simulink model "momentumBasedFlying"  (Simulink 10.2)
settings: Solver=FixedStepAuto  StartTime=0.0  StopTime=Config.simulationTime  FixedStep=Config.tStep  RelTol=1e-3
InitFcn:
  | cd(fileparts(which(bdroot)));
  | initMomentumBasedFlying;
StopFcn:
  | cd(fileparts(which(bdroot)));
  | stopMomentumBasedFlying;
undefined symbols (not defined in the file or in its folder): biasVectorConstraint_feet, Config, confVisualizer, ConstraintMatrix_feet, DiscIntNeverNeededParam, jets_config
libraries: WBToolboxLibrary x85
(part 2 of 4)

== system momentumBasedFlying/FLYING CONTROLLER (CORE) V2.5/Flying State Machine/Compute Gains And References ==
  joyAxes : Inport
  joyButtons : Inport  Port=2
  systemState : Inport  Port=3
  jointPos : Inport  Port=4
  stateMachineQuantities : Inport  Port=5
  Bus Creator : BusCreator  Inputs=8
  "CoM6D ->  CoMXYZ5" : Selector  NumberOfDimensions=2  InputPortWidth=7  IndexOptions=Index vector (dialog),Index vector (dialog)  Indices=[1 2 3],[1]  OutputSizes=1,1
  Compute Gains : Subsystem
  Constant : Constant  Value=Config.references.gainSmoothingRotation
  Constant1 : Constant  Value=Config.references.smoothingTimeCoM
  Smooth CoM and Base References : Subsystem
  To Workspace : ToWorkspace  VariableName=posCoM_int  SaveFormat=Timeseries  SampleTime=-1
  Trajectory Generator : Subsystem
  holder 2 : WBToolboxLibrary/Utilities/holder 
      settings: SourceProductName=WholeBodyToolbox
  gainsAndReferences : Outport  VectorParamsAs1DForOutWhenUnconnected=off
  tag scope: jointPos_des=global, posCoM_des=global, rot_vel_acc_jerk_base_des=global
  wires:
  "CoM6D ->  CoMXYZ5"/1 -> [posCoM_des]
  Constant1/1 -> Smooth CoM and Base References/2(smoothingTimeCoMPos)
  Smooth CoM and Base References/2(rot_vel_acc_jerk_base_des_smooth) -> [rot_vel_acc_jerk_base_des], Bus Creator/2  "rot_vel_acc_jerk_base_des"
  Compute Gains/5(KP_torqueControl) -> Bus Creator/8  "KP_torqueControl"
  Compute Gains/2(KD_momentum) -> Bus Creator/5  "KD_momentum"
  Compute Gains/1(KP_momentum) -> Bus Creator/4  "KP_momentum"
  Compute Gains/3(KP_postural) -> Bus Creator/6  "KP_postural"
  Constant/1 -> Smooth CoM and Base References/3(gainSmoothingBaseRot)
  Bus Creator/1 -> gainsAndReferences/1
  Compute Gains/4(KI_torqueControl) -> Bus Creator/7  "KI_torqueControl"
  holder 2/1 -> Bus Creator/1, [jointPos_des]  "jointPos_des"
  jointPos/1 -> holder 2/1
  joyAxes/1 -> Trajectory Generator/1(joyAxes)
  joyButtons/1 -> Trajectory Generator/2(joyButtons)
  systemState/1 -> Trajectory Generator/3(systemState)
  stateMachineQuantities/1 -> Trajectory Generator/4(stateMachineQuantities)
  Trajectory Generator/1(pos_vel_acc_jerk_CoM_des) -> Smooth CoM and Base References/1(pos_vel_acc_jerk_CoM_des)
  Trajectory Generator/2(rot_vel_acc_jerk_base_des) -> Smooth CoM and Base References/4(rot_vel_acc_jerk_base_des)
  Trajectory Generator/3(posCoM_int) -> To Workspace/1
  Smooth CoM and Base References/1(pos_vel_acc_jerk_CoM_des_smooth) -> "CoM6D ->  CoMXYZ5"/1, Bus Creator/3  "pos_vel_acc_jerk_CoM_des"

== system momentumBasedFlying/FLYING CONTROLLER (CORE) V2.5/Flying State Machine/Take Off/Landing State Detector ==
  systemState : Inport
  joyButtons : Inport  Port=2
  Bus Creator : BusCreator  Inputs=6
  Bus Selector : BusSelector  OutputSignals=contactForces
  Demux : Demux  Outputs=[6;6]
  MATLAB Function : MATLAB Function  TreatAsAtomicUnit=on
  Vertical Forces Control : MATLAB Function  TreatAsAtomicUnit=on
  stateMachineQuantities : Outport  VectorParamsAs1DForOutWhenUnconnected=off
  tag scope: stateMachineQuantities=global
  wires:
  Vertical Forces Control/1(decreaseMaxFootVerticalForce) -> Bus Creator/1  "decreaseMaxFootVerticalForce"
  Vertical Forces Control/2(increaseMinFootVerticalForce) -> Bus Creator/2  "increaseMinFootVerticalForce"
  Bus Creator/1 -> [stateMachineQuantities], stateMachineQuantities/1
  systemState/1 -> Bus Selector/1
  joyButtons/1 -> Vertical Forces Control/1(joyButtons)
  Demux/2 -> MATLAB Function/2(wrench_r)
  Demux/1 -> MATLAB Function/1(wrench_l)
  Bus Selector/1 -> Demux/1  "<contactForces>"
  MATLAB Function/1(feetContactIsActive) -> Bus Creator/4  "feetContactIsActive"
  MATLAB Function/2(robotIsLanded) -> Bus Creator/5  "robotIsLanded"
  MATLAB Function/3(oneFootIsInContact) -> Bus Creator/6  "oneFootIsInContact"
  Vertical Forces Control/3(activateEqConstrTorqueControl) -> Bus Creator/3  "activateEqConstrTorqueControl"

== system momentumBasedFlying/FLYING CONTROLLER (CORE) V2.5/Get System State/Change Contact Forces Representation ==
  jointPos : Inport
  w_H_b : Inport  Port=2
  contactForces_WBD : Inport  Port=3
  Change Contact Forces Representation : MATLAB Function  TreatAsAtomicUnit=on
  "CoM6D ->  CoMXYZ1" : Selector  NumberOfDimensions=2  InputPortWidth=7  IndexOptions=Index vector (dialog),Index vector (dialog)  Indices=[1 2 3],[1 2 3]  OutputSizes=1,1
  "CoM6D ->  CoMXYZ3" : Selector  NumberOfDimensions=2  InputPortWidth=7  IndexOptions=Index vector (dialog),Index vector (dialog)  Indices=[1 2 3],[1 2 3]  OutputSizes=1,1
  LFoot Pose : WBToolboxLibrary/Model/Kinematics/ForwardKinematics  frameName=Frames.LFOOT_FRAME
      settings: SourceProductName=WholeBodyToolbox
  Mux : Mux  Inputs=2
  RFoot Pose : WBToolboxLibrary/Model/Kinematics/ForwardKinematics  frameName=Frames.RFOOT_FRAME
      settings: SourceProductName=WholeBodyToolbox
  contactForces : Outport  VectorParamsAs1DForOutWhenUnconnected=off
  tag scope: wrench_LFoot=global, wrench_RFoot=global
  wires:
  contactForces_WBD/1 -> Change Contact Forces Representation/1(contactForces_WBD)
  RFoot Pose/1 -> "CoM6D ->  CoMXYZ3"/1
  "CoM6D ->  CoMXYZ3"/1 -> Change Contact Forces Representation/3(w_R_r_sole)
  LFoot Pose/1 -> "CoM6D ->  CoMXYZ1"/1
  "CoM6D ->  CoMXYZ1"/1 -> Change Contact Forces Representation/2(w_R_l_sole)
  w_H_b/1 -> LFoot Pose/1, RFoot Pose/1
  jointPos/1 -> LFoot Pose/2, RFoot Pose/2
  Change Contact Forces Representation/1(mixed_f_l_sole) -> [wrench_LFoot], Mux/1
  Change Contact Forces Representation/2(mixed_f_r_sole) -> [wrench_RFoot], Mux/2
  Mux/1 -> contactForces/1

== system momentumBasedFlying/Visualizer/Task and Base Frame Kinematics/Combine Rotations ==
  roll : Inport
  pitch : Inport  Port=2
  yaw : Inport  Port=3
  roll_des : Inport  Port=4
  pitch_des : Inport  Port=5
  yaw_des : Inport  Port=6
  Mux : Mux  Inputs=2
  Mux1 : Mux  Inputs=2
  Mux2 : Mux  Inputs=2
  Task rotation combined : Scope  NumInputPorts=3
  wires:
  yaw_des/1 -> Mux2/2
  pitch_des/1 -> Mux1/2
  pitch/1 -> Mux1/1
  roll/1 -> Mux/1
  yaw/1 -> Mux2/1
  roll_des/1 -> Mux/2
  Mux2/1 -> Task rotation combined/3
  Mux1/1 -> Task rotation combined/2
  Mux/1 -> Task rotation combined/1

== system momentumBasedFlying/iRonCub/Forward Dynamics/old_simulator_subsystem ==
  joints_torque : Inport
  systemState : Inport  Port=2
  jets_input : Inport  Port=3
  Bus Creator : BusCreator  Inputs=5
  Bus Selector : BusSelector  Commented=on  OutputSignals=M,h
  Bus Selector1 : BusSelector  OutputSignals=baseTwist,jointVelocity,J_LFoot,J_RFoot,JDot_LFoot_nu,JDot_RFoot_nu,w_H_LFoot,w_H_RFoot,w_R_b
  Compute generalized external wrench and jet thrust : Subsystem
  Dynamics and Kinematics : Subsystem
  MATLAB Function1 : MATLAB Function  TreatAsAtomicUnit=on
  State Integration : Subsystem
  state : Outport
  wrench_LFoot : Outport  Port=2
  wrench_RFoot : Outport  Port=3
  wires:
  State Integration/3(basePose_dot) -> Bus Creator/3
  Dynamics and Kinematics/2(kinematics) -> Compute generalized external wrench and jet thrust/1(kinematics), Bus Selector1/1  "kinematics"
  Bus Selector1/6 -> MATLAB Function1/10(JDot_nu_RFOOT)  "<JDot_RFoot_nu>"
  Bus Selector1/7 -> MATLAB Function1/11(H_LFOOT)  "<w_H_LFoot>"
  Bus Selector1/4 -> MATLAB Function1/8(JRight_frameJac)  "<J_RFoot>"
  Bus Selector1/3 -> MATLAB Function1/7(JLeft_frameJac)  "<J_LFoot>"
  MATLAB Function1/4(dot_v_b) -> State Integration/5(dot_v_b)
  Bus Selector1/2 -> MATLAB Function1/6("joints_velocity ")  "<jointVelocity>"
  Compute generalized external wrench and jet thrust/1(generalized_jet_wrench) -> MATLAB Function1/4(generalized_ext_wrench)
  Bus Creator/1 -> state/1  "state"
  State Integration/4("joints_velocity ") -> Bus Creator/4
  Dynamics and Kinematics/1(dynamics) -> Bus Selector/1
  joints_torque/1 -> MATLAB Function1/3(joints_torque)
  State Integration/2(joints_position) -> Bus Creator/2
  MATLAB Function1/8(wrench_left_foot) -> wrench_LFoot/1  "wrench_LFoot"
  jets_input/1 -> Compute generalized external wrench and jet thrust/2(jets_input)
  State Integration/1(w_H_b) -> Bus Creator/1
  Bus Selector1/8 -> MATLAB Function1/12(H_RFOOT)  "<w_H_RFoot>"
  systemState/1 -> Dynamics and Kinematics/1(systemState)
  Bus Selector1/9 -> State Integration/1(<w_R_b>)  "<w_R_b>"
  Compute generalized external wrench and jet thrust/2(jets_intensities) -> Bus Creator/5  "jet_intensities"
  MATLAB Function1/6(joint_acceleration) -> State Integration/7(joint_acceleration)
  MATLAB Function1/3(joints_velocity) -> State Integration/4(joints_velocity)
  MATLAB Function1/9(wrench_right_foot) -> wrench_RFoot/1  "wrench_RFoot"
  Bus Selector1/5 -> MATLAB Function1/9(JDot_nu_LFOOT)  "<JDot_LFoot_nu>"
  Bus Selector/1 -> MATLAB Function1/1(mass_matrix)  "<M>"
  MATLAB Function1/1(base_linear_velocity) -> State Integration/2(base_linear_velocity)
  Bus Selector/2 -> MATLAB Function1/2(bias_forces)  "<h>"
  MATLAB Function1/7(contact_detected) -> State Integration/8(contact_detected)
  MATLAB Function1/2(omega_b) -> State Integration/3(omega_b)
  Bus Selector1/1 -> MATLAB Function1/5(base_velocity)  "<baseTwist>"
  MATLAB Function1/5(dot_omega_b) -> State Integration/6(dot_omega_b)

== system momentumBasedFlying/FLYING CONTROLLER (CORE) V2.5/Dynamics and Kinematics/Dynamic Quantities/Compute Centroidal Inertia ==
  M : Inport
  w_H_b : Inport  Port=2
  posCoM : Inport  Port=3
  Compute Centroidal Inertia : MATLAB Function  TreatAsAtomicUnit=on
  Selector : Selector  NumberOfDimensions=2  InputPortWidth=3  IndexOptions=Index vector (dialog),Index vector (dialog)  Indices=[1 2 3],4  OutputSizes=1,1
  w_I_c : Outport  VectorParamsAs1DForOutWhenUnconnected=off
  wires:
  M/1 -> Compute Centroidal Inertia/1(M)
  w_H_b/1 -> Selector/1
  Selector/1 -> Compute Centroidal Inertia/3(posBase)
  posCoM/1 -> Compute Centroidal Inertia/2(posCoM)
  Compute Centroidal Inertia/1(w_I_c) -> w_I_c/1

== system momentumBasedFlying/FLYING CONTROLLER (CORE) V2.5/Dynamics and Kinematics/Dynamic Quantities/Momentum and CentroidalMomentum Matrix ==
  w_H_b : Inport
  jointPos : Inport  Port=2
  w_baseTwist : Inport  Port=3
  jointVel : Inport  Port=4
  CentroidalMomentum : WBToolboxLibrary/Model/Dynamics/CentroidalMomentum
      settings: SourceProductName=WholeBodyToolbox
  CentroidalMomentum Matrix iCub 23/25 DoFs : Subsystem
  L : Outport  VectorParamsAs1DForOutWhenUnconnected=off
  CMM : Outport  Port=2  VectorParamsAs1DForOutWhenUnconnected=off
  wires:
  w_baseTwist/1 -> CentroidalMomentum/3
  CentroidalMomentum/1 -> L/1
  w_H_b/1 -> CentroidalMomentum Matrix iCub 23/25 DoFs/1(w_H_b), CentroidalMomentum/1
  jointPos/1 -> CentroidalMomentum Matrix iCub 23/25 DoFs/2(jointPos), CentroidalMomentum/2
  jointVel/1 -> CentroidalMomentum/4
  CentroidalMomentum Matrix iCub 23/25 DoFs/1(CMM) -> CMM/1

== system momentumBasedFlying/FLYING CONTROLLER (CORE) V2.5/Dynamics and Kinematics/Kinematic Quantities/Compute Thrusts Axes and Arms ==
  posCoM : Inport
  w_H_b : Inport  Port=2
  jointPos : Inport  Port=3
  Pose Jet 1 : WBToolboxLibrary/Model/Kinematics/ForwardKinematics  frameName=Frames.JET1_FRAME
      settings: SourceProductName=WholeBodyToolbox
  Pose Jet 2 : WBToolboxLibrary/Model/Kinematics/ForwardKinematics  frameName=Frames.JET2_FRAME
      settings: SourceProductName=WholeBodyToolbox
  Pose Jet 3 : WBToolboxLibrary/Model/Kinematics/ForwardKinematics  frameName=Frames.JET3_FRAME
      settings: SourceProductName=WholeBodyToolbox
  Pose Jet 4 : WBToolboxLibrary/Model/Kinematics/ForwardKinematics  frameName=Frames.JET4_FRAME
      settings: SourceProductName=WholeBodyToolbox
  Thrust Axes and Arms : MATLAB Function  TreatAsAtomicUnit=on
  matrixOfJetsAxes : Outport  VectorParamsAs1DForOutWhenUnconnected=off
  matrixOfJetsArms : Outport  Port=2  VectorParamsAs1DForOutWhenUnconnected=off
  wires:
  Pose Jet 2/1 -> Thrust Axes and Arms/2(w_H_J2)
  jointPos/1 -> Pose Jet 1/2, Pose Jet 2/2, Pose Jet 3/2, Pose Jet 4/2
  Pose Jet 1/1 -> Thrust Axes and Arms/1(w_H_J1)
  Pose Jet 3/1 -> Thrust Axes and Arms/3(w_H_J3)
  Pose Jet 4/1 -> Thrust Axes and Arms/4(w_H_J4)
  Thrust Axes and Arms/1(matrixOfJetsAxes) -> matrixOfJetsAxes/1
  Thrust Axes and Arms/2(matrixOfJetsArms) -> matrixOfJetsArms/1
  w_H_b/1 -> Pose Jet 4/1, Pose Jet 3/1, Pose Jet 2/1, Pose Jet 1/1
  posCoM/1 -> Thrust Axes and Arms/5(posCoM)

== system momentumBasedFlying/FLYING CONTROLLER (CORE) V2.5/Flying Controller v2.5/Joint Torque Control for Flying/Integrate Joints Velocity error ==
  jointVel_err : Inport
  Constant : Constant  Value=zeros(Config.N_DOF,1)
  Discrete-Time Integrator1 : DiscreteIntegrator  InitialConditionSource=external  InitialCondition=zeros(Config.N_DOF,1)  SampleTime=-1  ICPrevOutput=DiscIntNeverNeededParam  ICPrevScaledInput=DiscIntNeverNeededParam
  jointPos_err : Outport  VectorParamsAs1DForOutWhenUnconnected=off
  tag scope: jointPos_err_integral=global
  wires:
  Discrete-Time Integrator1/1 -> jointPos_err/1, [jointPos_err_integral]
  jointVel_err/1 -> Discrete-Time Integrator1/1
  Constant/1 -> Discrete-Time Integrator1/2

== system momentumBasedFlying/FLYING CONTROLLER (CORE) V2.5/Flying Controller v2.5/Joint Torque Control for Flying/QP_torqueControl ==
  Hessian : Inport
  gradient : Inport  Port=2
  ConstraintMatrix_inequality : Inport  Port=3
  biasVectorConstraint_inequality : Inport  Port=4
  feetContactIsActive : Inport  Port=5
  Constant2 : Constant  Value=Config.sat.jointTorquesSaturation
  Level-2 MATLAB S-Function1 : M-S-Function  FunctionName=QP_flyingTorqueControl  Parameters=Config.N_DOF
  jointTorques_star : Outport  VectorParamsAs1DForOutWhenUnconnected=off
  exitFlagQP_torqueControl : Outport  Port=2  VectorParamsAs1DForOutWhenUnconnected=off
  wires:
  Hessian/1 -> Level-2 MATLAB S-Function1/1
  Level-2 MATLAB S-Function1/1 -> jointTorques_star/1
  gradient/1 -> Level-2 MATLAB S-Function1/2
  Level-2 MATLAB S-Function1/2 -> exitFlagQP_torqueControl/1
  Constant2/1 -> Level-2 MATLAB S-Function1/6
  ConstraintMatrix_inequality/1 -> Level-2 MATLAB S-Function1/3
  biasVectorConstraint_inequality/1 -> Level-2 MATLAB S-Function1/4
  feetContactIsActive/1 -> Level-2 MATLAB S-Function1/5

== system momentumBasedFlying/FLYING CONTROLLER (CORE) V2.5/Flying Controller v2.5/Joint Torque Control for Flying/Torque Derivative Saturation ==
  jointTorques_star : Inport
  Constant1 : Constant  Value=Config.tStep
  Constant2 : Constant  Value=Config.sat.jointTorquesDotMax
  Saturate Torque Derivative : MATLAB Function  TreatAsAtomicUnit=on
  "holder " : WBToolboxLibrary/Utilities/holder 
      settings: SourceProductName=WholeBodyToolbox
  jointTorques_star_sat : Outport  VectorParamsAs1DForOutWhenUnconnected=off
  wires:
  jointTorques_star/1 -> "holder "/1, Saturate Torque Derivative/1(u)
  Saturate Torque Derivative/1(uSat) -> jointTorques_star_sat/1
  "holder "/1 -> Saturate Torque Derivative/2(u_0)
  Constant1/1 -> Saturate Torque Derivative/3(tStep)
  Constant2/1 -> Saturate Torque Derivative/4(uDotMax)

== system momentumBasedFlying/FLYING CONTROLLER (CORE) V2.5/Flying Controller v2.5/Momentum Control for Flying/Feedback linearization ==
  jetState : Inport
  jetDerivatives_des : Inport  Port=2
  Bus Selector : BusSelector  OutputSignals=jetIntensitiesFiltered,jetDerivativesEst
  Discrete-Time Integrator : DiscreteIntegrator  SampleTime=Config.tStep  ICPrevOutput=DiscIntNeverNeededParam  ICPrevScaledInput=DiscIntNeverNeededParam
  Error : Scope
  MATLAB Function : MATLAB Function  TreatAsAtomicUnit=on
  jetDerivatives : Scope  NumInputPorts=3
  throttle : Outport  VectorParamsAs1DForOutWhenUnconnected=off
  wires:
  Bus Selector/1 -> MATLAB Function/1(jets)  "<jetIntensitiesFiltered>"
  MATLAB Function/1(throttle) -> jetDerivatives/1, throttle/1  "throttle"
  jetState/1 -> Bus Selector/1
  MATLAB Function/2(error) -> Error/1, Discrete-Time Integrator/1  "error"
  Bus Selector/2 -> jetDerivatives/3, MATLAB Function/2(jets_dot)  "<jetDerivativesEst>"
  Discrete-Time Integrator/1 -> MATLAB Function/4(integral_err)
  jetDerivatives_des/1 -> MATLAB Function/3(jets_dot_des), jetDerivatives/2

== system momentumBasedFlying/FLYING CONTROLLER (CORE) V2.5/Flying Controller v2.5/Momentum Control for Flying/Momentum Control ==
  contactForces_hat : Inport
  systemState : Inport  Port=2
  kinematics : Inport  Port=3
  dynamics : Inport  Port=4
  gainsAndReferences : Inport  Port=5
  stateMachineQuantitites : Inport  Port=6
  Bus Selector : BusSelector  OutputSignals=jointPos,w_baseTwist,jetsIntensities,contactForces
  Bus Selector1 : BusSelector  OutputSignals=J_jets,J_CoM,J_LFoot,J_RFoot,posCoM,w_R_b,w_H_LFoot,w_H_RFoot,matrixOfJetAxes,matrixOfJetsArms
  Bus Selector2 : BusSelector  OutputSignals=w_I_c,L,M,CMM
  Bus Selector3 : BusSelector  OutputSignals=pos_vel_acc_jerk_CoM_des,rot_vel_acc_jerk_base_des,jointPos_des,KP_momentum,KD_momentum,KP_postural
  Bus Selector4 : BusSelector  OutputSignals=feetContactIsActive,decreaseMaxFootVerticalForce,increaseMinFootVerticalForce,robotIsLanded
  "Flying Controller Momentum FCN " : MATLAB Function  TreatAsAtomicUnit=on
  HessianMatrixQP : Outport  VectorParamsAs1DForOutWhenUnconnected=off
  gVectorQP : Outport  Port=2  VectorParamsAs1DForOutWhenUnconnected=off
  lowerBoundQP : Outport  Port=3  VectorParamsAs1DForOutWhenUnconnected=off
  uppeBoundQP : Outport  Port=4  VectorParamsAs1DForOutWhenUnconnected=off
  tag scope: LDot_estimated=global, momentum_des=global, verifyAngMomAndInertia=global
  wires:
  systemState/1 -> Bus Selector/1
  Bus Selector3/3 -> "Flying Controller Momentum FCN "/20(jointPos_des)  "<jointPos_des>"
  Bus Selector1/3 -> "Flying Controller Momentum FCN "/6(J_LFoot)  "<J_LFoot>"
  kinematics/1 -> Bus Selector1/1
  Bus Selector/1 -> "Flying Controller Momentum FCN "/1(jointPos)  "<jointPos>"
  Bus Selector1/1 -> "Flying Controller Momentum FCN "/4(J_jets)  "<J_jets>"
  Bus Selector/2 -> "Flying Controller Momentum FCN "/2(w_baseTwist)  "<w_baseTwist>"
  "Flying Controller Momentum FCN "/1(HessianMatrixQP) -> HessianMatrixQP/1
  "Flying Controller Momentum FCN "/4(upperBoundQP) -> uppeBoundQP/1
  "Flying Controller Momentum FCN "/2(gVectorQP) -> gVectorQP/1
  Bus Selector4/1 -> "Flying Controller Momentum FCN "/24(feetContactIsActive)  "<feetContactIsActive>"
  "Flying Controller Momentum FCN "/7(verifyAngMomAndInertia) -> [verifyAngMomAndInertia]
  stateMachineQuantitites/1 -> Bus Selector4/1
  "Flying Controller Momentum FCN "/3(lowerBoundQP) -> lowerBoundQP/1
  Bus Selector3/4 -> "Flying Controller Momentum FCN "/21(KP_momentum)  "<KP_momentum>"
  dynamics/1 -> Bus Selector2/1
  Bus Selector1/2 -> "Flying Controller Momentum FCN "/5(J_CoM)  "<J_CoM>"
  gainsAndReferences/1 -> Bus Selector3/1
  Bus Selector/3 -> "Flying Controller Momentum FCN "/3(jetsIntensities)  "<jetsIntensities>"
  Bus Selector1/4 -> "Flying Controller Momentum FCN "/7(J_RFoot)  "<J_RFoot>"
  Bus Selector1/8 -> "Flying Controller Momentum FCN "/11(w_H_RFoot)  "<w_H_RFoot>"
  Bus Selector2/4 -> "Flying Controller Momentum FCN "/17(CMM)  "<CMM>"
  Bus Selector2/3 -> "Flying Controller Momentum FCN "/16(M)  "<M>"
  "Flying Controller Momentum FCN "/6(LDot_estimated) -> [LDot_estimated]
  Bus Selector3/5 -> "Flying Controller Momentum FCN "/22(KD_momentum)  "<KD_momentum>"
  Bus Selector1/7 -> "Flying Controller Momentum FCN "/10(w_H_LFoot)  "<w_H_LFoot>"
  Bus Selector2/2 -> "Flying Controller Momentum FCN "/15(L)  "<L>"
  Bus Selector3/6 -> "Flying Controller Momentum FCN "/23(KP_postural)  "<KP_postural>"
  "Flying Controller Momentum FCN "/5(L_des) -> [momentum_des]
  Bus Selector1/5 -> "Flying Controller Momentum FCN "/8(posCoM)  "<posCoM>"
  Bus Selector3/2 -> "Flying Controller Momentum FCN "/19(rot_vel_acc_jerk_base_des)  "<rot_vel_acc_jerk_base_des>"
  Bus Selector1/6 -> "Flying Controller Momentum FCN "/9(w_R_b)  "<w_R_b>"
  Bus Selector3/1 -> "Flying Controller Momentum FCN "/18(pos_vel_acc_jerk_CoM_des)  "<pos_vel_acc_jerk_CoM_des>"
  Bus Selector1/9 -> "Flying Controller Momentum FCN "/12(matrixOfJetsAxes)  "<matrixOfJetAxes>"
  Bus Selector1/10 -> "Flying Controller Momentum FCN "/13(matrixOfJetsArms)  "<matrixOfJetsArms>"
  Bus Selector2/1 -> "Flying Controller Momentum FCN "/14(w_I_c)  "<w_I_c>"
  Bus Selector4/2 -> "Flying Controller Momentum FCN "/25(decreaseMaxFootVerticalForce)  "<decreaseMaxFootVerticalForce>"
  Bus Selector4/3 -> "Flying Controller Momentum FCN "/26(increaseMinFootVerticalForce)  "<increaseMinFootVerticalForce>"
  Bus Selector4/4 -> "Flying Controller Momentum FCN "/27(robotIsLanded)  "<robotIsLanded>"
  Bus Selector/4 -> "Flying Controller Momentum FCN "/28(contactForces_hat)  "<contactForces>"

== system momentumBasedFlying/FLYING CONTROLLER (CORE) V2.5/Flying Controller v2.5/Momentum Control for Flying/QP Solver and Integrate Contact Forces Derivative ==
  HessianMatrixQP : Inport
  gVectorQP : Inport  Port=2
  lowerBoundQP : Inport  Port=3
  upperBoundQP : Inport  Port=4
  stateMachineQuantities : Inport  Port=5
  systemState : Inport  Port=6
  Bus Selector1 : BusSelector  OutputSignals=feetContactIsActive
  Bus Selector2 : BusSelector  OutputSignals=contactForces
  Integrate the Contact Forces Derivative : Subsystem
  Level-2 MATLAB S-Function1 : M-S-Function  FunctionName=QP_flyingMomentumControl  Parameters=Config.N_DOF
  contactForces_star : Outport  VectorParamsAs1DForOutWhenUnconnected=off
  jetsIntensitiesDot_star : Outport  Port=2  VectorParamsAs1DForOutWhenUnconnected=off
  jointVel_star : Outport  Port=3  VectorParamsAs1DForOutWhenUnconnected=off
  tag scope: contactForces_star=global, exitFlagQP_momentumControl=global, jetsIntensitiesDot_star=global, jointVel_star=global
  wires:
  Integrate the Contact Forces Derivative/1(contactForces_star) -> contactForces_star/1, [contactForces_star]
  Level-2 MATLAB S-Function1/2 -> Integrate the Contact Forces Derivative/1(contactForcesDot_star)
  lowerBoundQP/1 -> Level-2 MATLAB S-Function1/3
  upperBoundQP/1 -> Level-2 MATLAB S-Function1/4
  Level-2 MATLAB S-Function1/4 -> [exitFlagQP_momentumControl]
  gVectorQP/1 -> Level-2 MATLAB S-Function1/2
  stateMachineQuantities/1 -> Bus Selector1/1
  HessianMatrixQP/1 -> Level-2 MATLAB S-Function1/1
  Level-2 MATLAB S-Function1/1 -> jetsIntensitiesDot_star/1, [jetsIntensitiesDot_star]
  Level-2 MATLAB S-Function1/3 -> [jointVel_star], jointVel_star/1
  Bus Selector1/1 -> Integrate the Contact Forces Derivative/3(feetContactIsActive), Level-2 MATLAB S-Function1/5  "<feetContactIsActive>"
  Bus Selector2/1 -> Integrate the Contact Forces Derivative/2(contactForces)  "<contactForces>"
  systemState/1 -> Bus Selector2/1

== system momentumBasedFlying/FLYING CONTROLLER (CORE) V2.5/Flying Controller v2.5/Momentum Control for Flying/extendedKalmanFilter4jets ==
  "jetsIntensityMeasured " : Inport
  "jetsThrottle " : Inport  Port=2
  Bus Creator : BusCreator  Inputs=2
  Demux : Demux
  Demux1 : Demux
  EKF_jet1 : Subsystem
  EKF_jet2 : Subsystem
  EKF_jet3 : Subsystem
  EKF_jet4 : Subsystem
  Mux : Mux
  Mux1 : Mux
  jetsState : Outport
  wires:
  Demux/1 -> EKF_jet1/1(input)
  Demux/2 -> EKF_jet2/1(input)
  Demux/3 -> EKF_jet3/1(input)
  Demux/4 -> EKF_jet4/1(input)
  Demux1/1 -> EKF_jet1/2(jetIntensityMeasurement)
  Demux1/2 -> EKF_jet2/2(jetIntensityMeasurement)
  Demux1/3 -> EKF_jet3/2(jetIntensityMeasurement)
  Demux1/4 -> EKF_jet4/2(jetIntensityMeasurement)
  EKF_jet2/1(jetIntensityFiltered) -> Mux/2
  EKF_jet1/1(jetIntensityFiltered) -> Mux/1
  EKF_jet3/1(jetIntensityFiltered) -> Mux/3
  EKF_jet4/1(jetIntensityFiltered) -> Mux/4
  EKF_jet1/2(jetDerivativeEstimated) -> Mux1/1
  EKF_jet2/2(jetDerivativeEstimated) -> Mux1/2
  EKF_jet3/2(jetDerivativeEstimated) -> Mux1/3
  EKF_jet4/2(jetDerivativeEstimated) -> Mux1/4
  "jetsThrottle "/1 -> Demux/1
  "jetsIntensityMeasured "/1 -> Demux1/1
  Mux/1 -> Bus Creator/1  "jetIntensitiesFiltered"
  Mux1/1 -> Bus Creator/2  "jetDerivativesEst"
  Bus Creator/1 -> jetsState/1

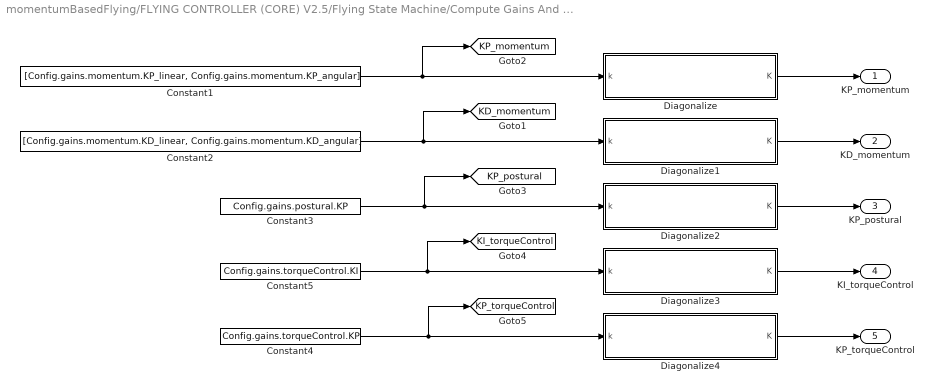
== system momentumBasedFlying/FLYING CONTROLLER (CORE) V2.5/Flying State Machine/Compute Gains And References/Compute Gains ==
  Constant1 : Constant  Value=[Config.gains.momentum.KP_linear, Config.gains.momentum.KP_angular]
  Constant2 : Constant  Value=[Config.gains.momentum.KD_linear, Config.gains.momentum.KD_angular]
  Constant3 : Constant  Value=Config.gains.postural.KP
  Constant4 : Constant  Value=Config.gains.torqueControl.KP
  Constant5 : Constant  Value=Config.gains.torqueControl.KI
  Diagonalize : MATLAB Function  TreatAsAtomicUnit=on
  Diagonalize1 : MATLAB Function  TreatAsAtomicUnit=on
  Diagonalize2 : MATLAB Function  TreatAsAtomicUnit=on
  Diagonalize3 : MATLAB Function  TreatAsAtomicUnit=on
  Diagonalize4 : MATLAB Function  TreatAsAtomicUnit=on
  KP_momentum : Outport  VectorParamsAs1DForOutWhenUnconnected=off
  KD_momentum : Outport  Port=2  VectorParamsAs1DForOutWhenUnconnected=off
  KP_postural : Outport  Port=3  VectorParamsAs1DForOutWhenUnconnected=off
  KI_torqueControl : Outport  Port=4  VectorParamsAs1DForOutWhenUnconnected=off
  KP_torqueControl : Outport  Port=5  VectorParamsAs1DForOutWhenUnconnected=off
  tag scope: KD_momentum=global, KI_torqueControl=global, KP_momentum=global, KP_postural=global, KP_torqueControl=global
  wires:
  Diagonalize/1(K) -> KP_momentum/1
  Diagonalize1/1(K) -> KD_momentum/1
  Diagonalize2/1(K) -> KP_postural/1
  Diagonalize3/1(K) -> KI_torqueControl/1
  Diagonalize4/1(K) -> KP_torqueControl/1
  Constant1/1 -> [KP_momentum], Diagonalize/1(k)
  Constant2/1 -> [KD_momentum], Diagonalize1/1(k)
  Constant3/1 -> [KP_postural], Diagonalize2/1(k)
  Constant5/1 -> [KI_torqueControl], Diagonalize3/1(k)
  Constant4/1 -> [KP_torqueControl], Diagonalize4/1(k)

== system momentumBasedFlying/FLYING CONTROLLER (CORE) V2.5/Flying State Machine/Compute Gains And References/Smooth CoM and Base References ==
  pos_vel_acc_jerk_CoM_des : Inport
  smoothingTimeCoMPos : Inport  Port=2
  gainSmoothingBaseRot : Inport  Port=3
  rot_vel_acc_jerk_base_des : Inport  Port=4
  Constant : Constant  Value=Config.references.SMOOTH_BASE_ROT_REFERENCES
  Constant1 : Constant  Value=Config.references.SMOOTH_COM_POS_REFERENCES
  Smooth Position References : Subsystem
  Smooth Reference Orientations : Subsystem
  Switch : Switch  Criteria=u2 > Threshold
  Switch2 : Switch  Criteria=u2 > Threshold
  pos_vel_acc_jerk_CoM_des_smooth : Outport  VectorParamsAs1DForOutWhenUnconnected=off
  rot_vel_acc_jerk_base_des_smooth : Outport  Port=2  VectorParamsAs1DForOutWhenUnconnected=off
  wires:
  Smooth Position References/1(pos_vel_acc_jerk_CoM_des_smooth) -> Switch/1
  smoothingTimeCoMPos/1 -> Smooth Position References/1(smoothingTimeCoMPos)
  pos_vel_acc_jerk_CoM_des/1 -> Switch/3, Smooth Position References/2(pos_vel_acc_jerk_CoM_des)
  Switch2/1 -> rot_vel_acc_jerk_base_des_smooth/1
  Switch/1 -> pos_vel_acc_jerk_CoM_des_smooth/1
  Constant1/1 -> Switch/2
  rot_vel_acc_jerk_base_des/1 -> Smooth Reference Orientations/1(rot_vel_acc_jerk_base_des)
  gainSmoothingBaseRot/1 -> Switch2/3, Smooth Reference Orientations/2(gainSmoothingBaseRot)
  Smooth Reference Orientations/1(rot_acc_vel_jerk_base_des_smooth) -> Switch2/1
  Constant/1 -> Switch2/2

== system momentumBasedFlying/FLYING CONTROLLER (CORE) V2.5/Flying State Machine/Compute Gains And References/Trajectory Generator ==
  joyAxes : Inport
  joyButtons : Inport  Port=2
  systemState : Inport  Port=3
  stateMachineQuantities : Inport  Port=4
  Bus Selector : BusSelector  OutputSignals=w_H_b,jointPos
  Bus Selector1 : BusSelector  OutputSignals=feetContactIsActive,oneFootIsInContact
  Clock : Clock
  Compute CoM and Base Rotation References : MATLAB Function  TreatAsAtomicUnit=on
  Detect Robot Movement Request From Joystick : MATLAB Function  TreatAsAtomicUnit=on
  ForwardKinematics : WBToolboxLibrary/Model/Kinematics/ForwardKinematics  frameName=Frames.COM_FRAME
      settings: SourceProductName=WholeBodyToolbox
  Selector : Selector  NumberOfDimensions=2  InputPortWidth=3  IndexOptions=Index vector (dialog),Index vector (dialog)  Indices=[1 2 3],[1 2 3]  OutputSizes=1,1
  Selector1 : Selector  NumberOfDimensions=2  InputPortWidth=3  IndexOptions=Index vector (dialog),Index vector (dialog)  Indices=[1 2 3],[4]  OutputSizes=1,1
  "holder " : WBToolboxLibrary/Utilities/holder 
      settings: SourceProductName=WholeBodyToolbox
  holder 1 : WBToolboxLibrary/Utilities/holder 
      settings: SourceProductName=WholeBodyToolbox
  pos_vel_acc_jerk_CoM_des : Outport  VectorParamsAs1DForOutWhenUnconnected=off
  rot_vel_acc_jerk_base_des : Outport  Port=2  VectorParamsAs1DForOutWhenUnconnected=off
  posCoM_int : Outport  Port=3
  wires:
  Bus Selector1/2 -> Compute CoM and Base Rotation References/12(oneFootIsInContact)  "<oneFootIsInContact>"
  Detect Robot Movement Request From Joystick/8(goLandingPos) -> Compute CoM and Base Rotation References/10(goLandingPos)
  Selector1/1 -> posCoM_int/1, Compute CoM and Base Rotation References/1(posCoM_init)
  Compute CoM and Base Rotation References/2(rot_vel_acc_jerk_base_des) -> rot_vel_acc_jerk_base_des/1
  joyButtons/1 -> Detect Robot Movement Request From Joystick/2(joyButtons)
  joyAxes/1 -> Detect Robot Movement Request From Joystick/1(joyAxes)
  systemState/1 -> Bus Selector/1
  Clock/1 -> Compute CoM and Base Rotation References/13(t)
  Detect Robot Movement Request From Joystick/6(rotateYaw) -> Compute CoM and Base Rotation References/8(rotateYaw)
  Compute CoM and Base Rotation References/1(pos_vel_acc_jerk_CoM_des) -> pos_vel_acc_jerk_CoM_des/1
  Detect Robot Movement Request From Joystick/4(rotateRoll) -> Compute CoM and Base Rotation References/6(rotateRoll)
  ForwardKinematics/1 -> "holder "/1
  holder 1/1 -> Compute CoM and Base Rotation References/2(w_R_b_init)
  Bus Selector/1 -> Selector/1, ForwardKinematics/1  "<w_H_b>"
  Selector/1 -> holder 1/1
  Bus Selector1/1 -> Compute CoM and Base Rotation References/11(feetContactIsActive)  "<feetContactIsActive>"
  Detect Robot Movement Request From Joystick/5(rotatePitch) -> Compute CoM and Base Rotation References/7(rotatePitch)
  stateMachineQuantities/1 -> Bus Selector1/1
  Detect Robot Movement Request From Joystick/2(moveLateral) -> Compute CoM and Base Rotation References/4(moveLateral)
  Detect Robot Movement Request From Joystick/3(moveUpDown) -> Compute CoM and Base Rotation References/5(moveUpDown)
  Bus Selector/2 -> ForwardKinematics/2  "<jointPos>"
  "holder "/1 -> Selector1/1
  Detect Robot Movement Request From Joystick/1(moveFront) -> Compute CoM and Base Rotation References/3(moveFront)
  Detect Robot Movement Request From Joystick/7(turbo_mode) -> Compute CoM and Base Rotation References/9(turbo_mode)

== system momentumBasedFlying/iRonCub/Forward Dynamics/old_simulator_subsystem/Compute generalized external wrench and jet thrust ==
  kinematics : Inport
  jets_input : Inport  Port=2
  Bus Selector3 : BusSelector  OutputSignals=J_jets,matrixOfJetsAxes
  Compute generalized jet wrench : Subsystem
  Sum1 : Sum
  "thrust Gaussian noise " : RandomNumber  Variance=Config.thrust_noise
  generalized_jet_wrench : Outport
  jets_intensities : Outport  Port=2  VectorParamsAs1DForOutWhenUnconnected=off
  wires:
  Sum1/1 -> jets_intensities/1  "jets_intensities"
  Bus Selector3/2 -> Compute generalized jet wrench/2(<matrixOfJetAxes>)  "<matrixOfJetsAxes>"
  jets_input/1 -> Compute generalized jet wrench/3(jets_input)
  Bus Selector3/1 -> Compute generalized jet wrench/1(<J_jets>)  "<J_jets>"
  kinematics/1 -> Bus Selector3/1
  "thrust Gaussian noise "/1 -> Sum1/1
  Compute generalized jet wrench/2(jet_intensities) -> Sum1/2  "jets_intensities"
  Compute generalized jet wrench/1(generalized_jet_wrench) -> generalized_jet_wrench/1

== system momentumBasedFlying/iRonCub/Forward Dynamics/old_simulator_subsystem/Dynamics and Kinematics ==
  systemState : Inport
  Bus Creator1 : BusCreator  Inputs=2
  Bus Creator2 : BusCreator  Inputs=16
  Bus Selector : BusSelector  OutputSignals=w_H_b,basePose_dot,joints_position,joints_velocity
  Dynamic Quantities : Subsystem
  Kinematic Quantities : Subsystem
  dynamics : Outport  VectorParamsAs1DForOutWhenUnconnected=off
  kinematics : Outport  Port=2  VectorParamsAs1DForOutWhenUnconnected=off
  wires:
  systemState/1 -> Bus Selector/1
  Bus Selector/1 -> Dynamic Quantities/1(w_H_b), Kinematic Quantities/1(w_H_b)  "<w_H_b>"
  Bus Selector/3 -> Dynamic Quantities/3(jointPos), Kinematic Quantities/3(jointPos)  "<joints_position>"
  Dynamic Quantities/2("h ") -> Bus Creator1/2  "h"
  Dynamic Quantities/1(M) -> Bus Creator1/1  "M"
  Bus Creator1/1 -> dynamics/1
  Bus Creator2/1 -> kinematics/1
  Kinematic Quantities/1(J_CoM) -> Bus Creator2/1  "J_CoM"
  Kinematic Quantities/2(w_R_b) -> Bus Creator2/2  "w_R_b"
  Kinematic Quantities/3(J_LFoot) -> Bus Creator2/3  "J_LFoot"
  Kinematic Quantities/4(J_RFoot) -> Bus Creator2/4  "J_RFoot"
  Kinematic Quantities/5(JDot_LFoot_nu) -> Bus Creator2/5  "JDot_LFoot_nu"
  Kinematic Quantities/6(JDot_RFoot_nu) -> Bus Creator2/6  "JDot_RFoot_nu"
  Kinematic Quantities/7(w_H_LFoot) -> Bus Creator2/7  "w_H_LFoot"
  Kinematic Quantities/8(w_H_RFoot) -> Bus Creator2/8  "w_H_RFoot"
  Kinematic Quantities/9(posCoM) -> Bus Creator2/9  "posCoM"
  Bus Selector/2 -> Kinematic Quantities/2(w_baseTwist), Dynamic Quantities/2(w_baseTwist)  "<basePose_dot>"
  Bus Selector/4 -> Kinematic Quantities/4(jointVel), Dynamic Quantities/4(jointVel)  "<joints_velocity>"
  Kinematic Quantities/11(baseTwist) -> Bus Creator2/11  "baseTwist"
  Kinematic Quantities/13(jointVelocity) -> Bus Creator2/13  "jointVelocity"
  Kinematic Quantities/10(wHb) -> Bus Creator2/10  "w_H_b"
  Kinematic Quantities/12(joint_pos) -> Bus Creator2/12  "jointPos"
  Kinematic Quantities/14(J_jets) -> Bus Creator2/14  "J_jets"
  Kinematic Quantities/15(matrixOfJetsAxes) -> Bus Creator2/15  "matrixOfJetsAxes"
  Kinematic Quantities/16(matrixOfJetsArms) -> Bus Creator2/16  "matrixOfJetsArms"

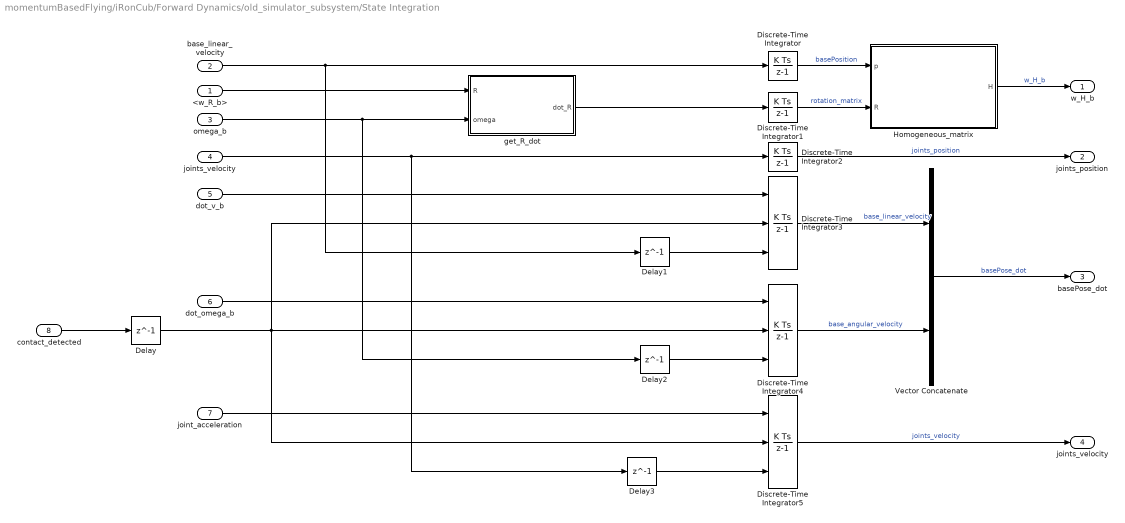
== system momentumBasedFlying/iRonCub/Forward Dynamics/old_simulator_subsystem/State Integration ==
  <w_R_b> : Inport
  base_linear_velocity : Inport  Port=2
  omega_b : Inport  Port=3
  joints_velocity : Inport  Port=4
  dot_v_b : Inport  Port=5
  dot_omega_b : Inport  Port=6
  joint_acceleration : Inport  Port=7
  contact_detected : Inport  Port=8
  Delay : Delay  DelayLength=1  InitialCondition=0
  Delay1 : Delay  DelayLength=1  InitialCondition=Config.initialConditions.base_linear_velocity
  Delay2 : Delay  DelayLength=1  InitialCondition=Config.initialConditions.base_angular_velocity
  Delay3 : Delay  DelayLength=1  InitialCondition=Config.initialConditions.joints_velocity
  Discrete-Time Integrator : DiscreteIntegrator  InitialCondition=Config.initialConditions.base_position  SampleTime=-1  ICPrevOutput=DiscIntNeverNeededParam  ICPrevScaledInput=DiscIntNeverNeededParam
  Discrete-Time Integrator1 : DiscreteIntegrator  InitialCondition=Config.initialConditions.orientation  SampleTime=-1  ICPrevOutput=DiscIntNeverNeededParam  ICPrevScaledInput=DiscIntNeverNeededParam
  Discrete-Time Integrator2 : DiscreteIntegrator  InitialCondition=Config.initialConditions.joints  SampleTime=-1  ICPrevOutput=DiscIntNeverNeededParam  ICPrevScaledInput=DiscIntNeverNeededParam
  Discrete-Time Integrator3 : DiscreteIntegrator  ExternalReset=rising  InitialConditionSource=external  InitialCondition=Config.initialConditions.base_linear_velocity  SampleTime=-1  ICPrevOutput=DiscIntNeverNeededParam  ICPrevScaledInput=DiscIntNeverNeededParam
  Discrete-Time Integrator4 : DiscreteIntegrator  ExternalReset=rising  InitialConditionSource=external  InitialCondition=Config.initialConditions.base_angular_velocity  SampleTime=-1  ICPrevOutput=DiscIntNeverNeededParam  ICPrevScaledInput=DiscIntNeverNeededParam
  Discrete-Time Integrator5 : DiscreteIntegrator  ExternalReset=rising  InitialConditionSource=external  InitialCondition=Config.initialConditions.joints_velocity  SampleTime=-1  ICPrevOutput=DiscIntNeverNeededParam  ICPrevScaledInput=DiscIntNeverNeededParam
  "Homogeneous_matrix " : MATLAB Function  TreatAsAtomicUnit=on
  Vector Concatenate : Concatenate
  "get_R_dot " : MATLAB Function  TreatAsAtomicUnit=on
  w_H_b : Outport  VectorParamsAs1DForOutWhenUnconnected=off
  joints_position : Outport  Port=2  VectorParamsAs1DForOutWhenUnconnected=off
  basePose_dot : Outport  Port=3  VectorParamsAs1DForOutWhenUnconnected=off
  "joints_velocity " : Outport  Port=4  VectorParamsAs1DForOutWhenUnconnected=off
  wires:
  Discrete-Time Integrator3/1 -> Vector Concatenate/1  "base_linear_velocity"
  omega_b/1 -> "get_R_dot "/2(omega), Delay2/1
  Discrete-Time Integrator5/1 -> "joints_velocity "/1  "joints_velocity"
  dot_v_b/1 -> Discrete-Time Integrator3/1
  Discrete-Time Integrator2/1 -> joints_position/1  "joints_position"
  <w_R_b>/1 -> "get_R_dot "/1(R)
  Discrete-Time Integrator4/1 -> Vector Concatenate/2  "base_angular_velocity"
  "Homogeneous_matrix "/1(H) -> w_H_b/1  "w_H_b"
  Vector Concatenate/1 -> basePose_dot/1  "basePose_dot"
  joints_velocity/1 -> Discrete-Time Integrator2/1, Delay3/1
  Discrete-Time Integrator/1 -> "Homogeneous_matrix "/1(p)  "basePosition"
  "get_R_dot "/1(dot_R) -> Discrete-Time Integrator1/1
  dot_omega_b/1 -> Discrete-Time Integrator4/1
  joint_acceleration/1 -> Discrete-Time Integrator5/1
  Discrete-Time Integrator1/1 -> "Homogeneous_matrix "/2(R)  "rotation_matrix"
  base_linear_velocity/1 -> Discrete-Time Integrator/1, Delay1/1
  contact_detected/1 -> Delay/1
  Delay/1 -> Discrete-Time Integrator3/2, Discrete-Time Integrator4/2, Discrete-Time Integrator5/2
  Delay1/1 -> Discrete-Time Integrator3/3
  Delay2/1 -> Discrete-Time Integrator4/3
  Delay3/1 -> Discrete-Time Integrator5/3

== system momentumBasedFlying/FLYING CONTROLLER (CORE) V2.5/Dynamics and Kinematics/Dynamic Quantities/Momentum and CentroidalMomentum Matrix/CentroidalMomentum Matrix iCub 23/25 DoFs ==
  note: REQUIRED WORKSPACE PARAMETER:
      |
      | - Config.N_DOF: number of DoFs. Expected
      | values: either 23 or 25.
  w_H_b : Inport
  jointPos : Inport  Port=2
  CMM_base : Subsystem
  CMM_joints : Subsystem
  Combine CMM : Subsystem
  Constant : Constant  Value=eye(Config.N_DOF)
  Constant1 : Constant  Value=Config.N_DOF
  Constant2 : Constant  Value=Config.N_DOF
  Select CMM 23 or 25 : MATLAB Function  TreatAsAtomicUnit=on
  Selector Matrix : MATLAB Function  TreatAsAtomicUnit=on
  CMM : Outport  VectorParamsAs1DForOutWhenUnconnected=off
  wires:
  jointPos/1 -> CMM_base/2(jointPos), CMM_joints/2(jointPos)
  w_H_b/1 -> CMM_base/1(w_H_b), CMM_joints/1(w_H_b)
  Selector Matrix/1(SelMatrix) -> CMM_joints/3(SelMatrix)
  Constant1/1 -> Selector Matrix/1(ROBOT_DOF)
  Constant/1 -> Selector Matrix/2(SelMatrix_0)
  Combine CMM/1(CMM_25DoFs) -> Select CMM 23 or 25/1(CMM_25)
  CMM_base/1(CMM_base) -> Combine CMM/1(CMM_base)
  CMM_joints/1(CMM_joints_from_1_to_20) -> Combine CMM/2(CMM_joints_1_20)
  CMM_joints/2(CMM_group5_25DoFs) -> Combine CMM/3(CMM_group5_25DoFs)
  CMM_joints/3(CMM_group5_23DoFs) -> Combine CMM/4(CMM_group5_23DoFs)
  Constant2/1 -> Select CMM 23 or 25/2(N_DOF)
  Select CMM 23 or 25/1(CMM) -> CMM/1
  Combine CMM/2(CMM_23DoFs) -> Select CMM 23 or 25/3(CMM_23)

== system momentumBasedFlying/FLYING CONTROLLER (CORE) V2.5/Flying Controller v2.5/Momentum Control for Flying/QP Solver and Integrate Contact Forces Derivative/Integrate the Contact Forces Derivative ==
  contactForcesDot_star : Inport
  contactForces : Inport  Port=2
  feetContactIsActive : Inport  Port=3
  Discrete-Time Integrator1 : DiscreteIntegrator  ExternalReset=either  InitialConditionSource=external  InitialCondition=zeros(6,1)  SampleTime=Config.tStep  ICPrevOutput=DiscIntNeverNeededParam  ICPrevScaledInput=DiscIntNeverNeededParam
  Select Integrator Initial Condition : MATLAB Function  TreatAsAtomicUnit=on
  deadZone : Subsystem
  contactForces_star : Outport  VectorParamsAs1DForOutWhenUnconnected=off
  tag scope: contactForcesDot_star=global
  wires:
  Discrete-Time Integrator1/1 -> contactForces_star/1
  contactForcesDot_star/1 -> deadZone/1(u), [contactForcesDot_star]
  deadZone/1(u_cut) -> Discrete-Time Integrator1/1
  contactForces/1 -> Select Integrator Initial Condition/2(contactForces)
  feetContactIsActive/1 -> Select Integrator Initial Condition/1(feetContactIsActive), Discrete-Time Integrator1/2
  Select Integrator Initial Condition/1(contactForces_0) -> Discrete-Time Integrator1/3

== system momentumBasedFlying/FLYING CONTROLLER (CORE) V2.5/Flying Controller v2.5/Momentum Control for Flying/extendedKalmanFilter4jets/EKF_jet1 ==
  input : Inport
  jetIntensityMeasurement : Inport  Port=2
  Constant : Constant  Value=[Config.initT, Config.initTdot]
  Constant1 : Constant  Value=Config.ekf.initP
  Discrete-Time Integrator1 : DiscreteIntegrator  InitialConditionSource=external  SampleTime=Config.tStep  ICPrevOutput=DiscIntNeverNeededParam  ICPrevScaledInput=DiscIntNeverNeededParam
  Discrete-Time Integrator2 : DiscreteIntegrator  InitialConditionSource=external  SampleTime=Config.tStep  ICPrevOutput=DiscIntNeverNeededParam  ICPrevScaledInput=DiscIntNeverNeededParam
  "EKF " : MATLAB Function  TreatAsAtomicUnit=on
  splitVector : MATLAB Function  TreatAsAtomicUnit=on
  jetIntensityFiltered : Outport  VectorParamsAs1DForOutWhenUnconnected=off
  jetDerivativeEstimated : Outport  Port=2  VectorParamsAs1DForOutWhenUnconnected=off
  wires:
  splitVector/2(x2) -> jetDerivativeEstimated/1
  splitVector/1(x1) -> jetIntensityFiltered/1
  Constant1/1 -> Discrete-Time Integrator2/2
  Discrete-Time Integrator2/1 -> "EKF "/4(P)
  jetIntensityMeasurement/1 -> "EKF "/3(measurement)
  Constant/1 -> Discrete-Time Integrator1/2
  Discrete-Time Integrator1/1 -> splitVector/1(x), "EKF "/1(x)
  input/1 -> "EKF "/2(input)
  "EKF "/1(xDot) -> Discrete-Time Integrator1/1
  "EKF "/2(Pdot) -> Discrete-Time Integrator2/1

== system momentumBasedFlying/FLYING CONTROLLER (CORE) V2.5/Flying Controller v2.5/Momentum Control for Flying/extendedKalmanFilter4jets/EKF_jet2 ==
  input : Inport
  jetIntensityMeasurement : Inport  Port=2
  Constant : Constant  Value=[Config.initT, Config.initTdot]
  Constant1 : Constant  Value=Config.ekf.initP
  Discrete-Time Integrator1 : DiscreteIntegrator  InitialConditionSource=external  SampleTime=Config.tStep  ICPrevOutput=DiscIntNeverNeededParam  ICPrevScaledInput=DiscIntNeverNeededParam
  Discrete-Time Integrator2 : DiscreteIntegrator  InitialConditionSource=external  SampleTime=Config.tStep  ICPrevOutput=DiscIntNeverNeededParam  ICPrevScaledInput=DiscIntNeverNeededParam
  "EKF " : MATLAB Function  TreatAsAtomicUnit=on
  splitVector : MATLAB Function  TreatAsAtomicUnit=on
  jetIntensityFiltered : Outport  VectorParamsAs1DForOutWhenUnconnected=off
  jetDerivativeEstimated : Outport  Port=2  VectorParamsAs1DForOutWhenUnconnected=off
  wires:
  "EKF "/2(Pdot) -> Discrete-Time Integrator2/1
  "EKF "/1(xDot) -> Discrete-Time Integrator1/1
  input/1 -> "EKF "/2(input)
  Discrete-Time Integrator1/1 -> "EKF "/1(x), splitVector/1(x)
  Constant/1 -> Discrete-Time Integrator1/2
  jetIntensityMeasurement/1 -> "EKF "/3(measurement)
  Discrete-Time Integrator2/1 -> "EKF "/4(P)
  Constant1/1 -> Discrete-Time Integrator2/2
  splitVector/1(x1) -> jetIntensityFiltered/1
  splitVector/2(x2) -> jetDerivativeEstimated/1

== system momentumBasedFlying/FLYING CONTROLLER (CORE) V2.5/Flying Controller v2.5/Momentum Control for Flying/extendedKalmanFilter4jets/EKF_jet3 ==
  input : Inport
  jetIntensityMeasurement : Inport  Port=2
  Constant : Constant  Value=[Config.initT, Config.initTdot]
  Constant1 : Constant  Value=Config.ekf.initP
  Discrete-Time Integrator1 : DiscreteIntegrator  InitialConditionSource=external  SampleTime=Config.tStep  ICPrevOutput=DiscIntNeverNeededParam  ICPrevScaledInput=DiscIntNeverNeededParam
  Discrete-Time Integrator2 : DiscreteIntegrator  InitialConditionSource=external  SampleTime=Config.tStep  ICPrevOutput=DiscIntNeverNeededParam  ICPrevScaledInput=DiscIntNeverNeededParam
  "EKF " : MATLAB Function  TreatAsAtomicUnit=on
  splitVector : MATLAB Function  TreatAsAtomicUnit=on
  jetIntensityFiltered : Outport  VectorParamsAs1DForOutWhenUnconnected=off
  jetDerivativeEstimated : Outport  Port=2  VectorParamsAs1DForOutWhenUnconnected=off
  wires:
  splitVector/2(x2) -> jetDerivativeEstimated/1
  splitVector/1(x1) -> jetIntensityFiltered/1
  Constant1/1 -> Discrete-Time Integrator2/2
  Discrete-Time Integrator2/1 -> "EKF "/4(P)
  jetIntensityMeasurement/1 -> "EKF "/3(measurement)
  Constant/1 -> Discrete-Time Integrator1/2
  Discrete-Time Integrator1/1 -> splitVector/1(x), "EKF "/1(x)
  input/1 -> "EKF "/2(input)
  "EKF "/1(xDot) -> Discrete-Time Integrator1/1
  "EKF "/2(Pdot) -> Discrete-Time Integrator2/1

== system momentumBasedFlying/FLYING CONTROLLER (CORE) V2.5/Flying Controller v2.5/Momentum Control for Flying/extendedKalmanFilter4jets/EKF_jet4 ==
  input : Inport
  jetIntensityMeasurement : Inport  Port=2
  Constant : Constant  Value=[Config.initT, Config.initTdot]
  Constant1 : Constant  Value=Config.ekf.initP
  Discrete-Time Integrator1 : DiscreteIntegrator  InitialConditionSource=external  SampleTime=Config.tStep  ICPrevOutput=DiscIntNeverNeededParam  ICPrevScaledInput=DiscIntNeverNeededParam
  Discrete-Time Integrator2 : DiscreteIntegrator  InitialConditionSource=external  SampleTime=Config.tStep  ICPrevOutput=DiscIntNeverNeededParam  ICPrevScaledInput=DiscIntNeverNeededParam
  "EKF " : MATLAB Function  TreatAsAtomicUnit=on
  splitVector : MATLAB Function  TreatAsAtomicUnit=on
  jetIntensityFiltered : Outport  VectorParamsAs1DForOutWhenUnconnected=off
  jetDerivativeEstimated : Outport  Port=2  VectorParamsAs1DForOutWhenUnconnected=off
  wires:
  "EKF "/2(Pdot) -> Discrete-Time Integrator2/1
  "EKF "/1(xDot) -> Discrete-Time Integrator1/1
  input/1 -> "EKF "/2(input)
  Discrete-Time Integrator1/1 -> "EKF "/1(x), splitVector/1(x)
  Constant/1 -> Discrete-Time Integrator1/2
  jetIntensityMeasurement/1 -> "EKF "/3(measurement)
  Discrete-Time Integrator2/1 -> "EKF "/4(P)
  Constant1/1 -> Discrete-Time Integrator2/2
  splitVector/1(x1) -> jetIntensityFiltered/1
  splitVector/2(x2) -> jetDerivativeEstimated/1

== system momentumBasedFlying/FLYING CONTROLLER (CORE) V2.5/Flying State Machine/Compute Gains And References/Smooth CoM and Base References/Smooth Position References ==
  smoothingTimeCoMPos : Inport
  pos_vel_acc_jerk_CoM_des : Inport  Port=2
  "CoM6D ->  CoMXYZ5" : Selector  NumberOfDimensions=2  InputPortWidth=7  IndexOptions=Index vector (dialog),Index vector (dialog)  Indices=[1 2 3],[1]  OutputSizes=1,1
  Compute Smooth Jerk Reference : WBToolboxLibrary/Utilities/MinimumJerkTrajectoryGenerator  externalSettlingTime=off  settlingTime=Config.references.com.tSmoothingCoMAcc  sampleTime=Config.tStep  resetOnSettlingTime=off  firstDerivatives=on  secondDerivatives=off  explicitInitialValue=off
      settings: SourceProductName=WholeBodyToolbox
  Matrix Concatenate : Concatenate  NumInputs=4  Mode=Multidimensional array  ConcatenateDimension=2
  MinimumJerkTrajectoryGenerator : WBToolboxLibrary/Utilities/MinimumJerkTrajectoryGenerator  externalSettlingTime=on  settlingTime=3  sampleTime=Config.tStep  resetOnSettlingTime=off  firstDerivatives=on  secondDerivatives=on  explicitInitialValue=off
      settings: SourceProductName=WholeBodyToolbox
  Terminator : Terminator
  pos_vel_acc_jerk_CoM_des_smooth : Outport  VectorParamsAs1DForOutWhenUnconnected=off
  wires:
  pos_vel_acc_jerk_CoM_des/1 -> "CoM6D ->  CoMXYZ5"/1
  smoothingTimeCoMPos/1 -> MinimumJerkTrajectoryGenerator/2
  MinimumJerkTrajectoryGenerator/1 -> Matrix Concatenate/1
  Matrix Concatenate/1 -> pos_vel_acc_jerk_CoM_des_smooth/1
  "CoM6D ->  CoMXYZ5"/1 -> MinimumJerkTrajectoryGenerator/1
  MinimumJerkTrajectoryGenerator/2 -> Matrix Concatenate/2
  MinimumJerkTrajectoryGenerator/3 -> Matrix Concatenate/3, Compute Smooth Jerk Reference/1
  Compute Smooth Jerk Reference/1 -> Terminator/1
  Compute Smooth Jerk Reference/2 -> Matrix Concatenate/4
